simulink model "sim_motor"  (R2022b)
settings: Solver=VariableStepAuto  StartTime=0.0  StopTime=3  RelTol=1e-3
libraries: spsControlledVoltageSourceLib x1, spsDCMachineLib x1, spsDCVoltageSourceLib x1, fuzblock x1, spspowerguiLib x1
settings Model: Creator=alwal  LastModifiedBy=alwal
settings DataIOCC: SaveOutput=off  SaveTime=off  ReturnWorkspaceOutputs=off

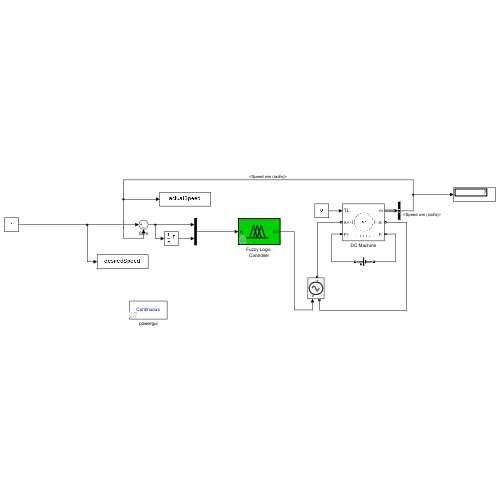
[thumbnail: Simulink's stored preview of the top-level diagram]
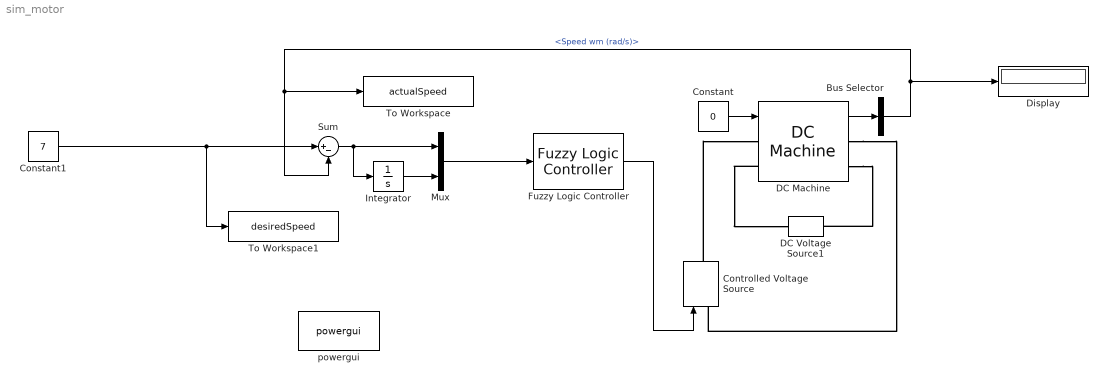
== system sim_motor ==
  Bus Selector : BusSelector  OutputSignals=Speed wm (rad/s)
  Constant : Constant  Value=0
  Constant1 : Constant  Value=7
  Controlled Voltage Source : spsControlledVoltageSourceLib/Controlled Voltage Source  Initialize=off  Source_Type=DC  Amplitude=0  Phase=0  Frequency=0  Measurements=Voltage
  DC Machine : spsDCMachineLib/DC Machine  PresetModel=No  MechanicalLoad=Torque TL  FieldType=Wound  ShowDetailedParameters=on  MeasurementBus=off  RLa="[ 0.6  0.012]"  RLf="[ 240  120]"  Laf=1.8  MachineConstant=Torque constant (N.m/A)  Ke=1.8  Kt=1.8  J=1  Bm=0  Tf=0  w0=1  Ifinit=0.0833333333333333  TsPowergui=0  TsBlock=-1
  DC Voltage Source1 : spsDCVoltageSourceLib/DC Voltage Source  Amplitude=20  Measurements=Voltage
  Display : Display
  Fuzzy Logic Controller : fuzblock/Fuzzy Logic  Controller  FIS=CLF02  OutputSampleNumber=101  DataType=double  FuzzifiedInputs=off  RuleFiringStrengths=off  RuleOutputs=off  AggregatedOutputs=off  SimulateUsing=Interpreted execution  OutOfRangeInputValueMessage=none  NoRuleFiredMessage=none  EmptyOutputFuzzySetMessage=none
  Integrator : Integrator  LimitOutput=on  UpperSaturationLimit=[9.7]  LowerSaturationLimit=[-9.7]
  Mux : Mux  Inputs=2
  Sum : Sum  Inputs=|+-
  To Workspace : ToWorkspace  VariableName=actualSpeed  SaveFormat=Timeseries
  To Workspace1 : ToWorkspace  VariableName=desiredSpeed  SaveFormat=Timeseries
  powergui : spspowerguiLib/powergui  Priority=1  SimulationMode=Continuous  SampleTime=50e-6  frequency=60  Iterations=50  frequencyindice=0  Pbase=100e6  ErrMax=1e-4  UnitsV=kV  UnitsW=MW  buscounter=0  FunctionMessages=off  echomessages=off  EnableUseOfTLC=off  CurrentSourceSwitches=off  DisableSnubberDevices=off  DisableRonSwitches=off  DisableVfSwitches=off  DisplayEquations=off  AutomaticDiscreteSolvers=off  SolverType=Tustin/Backward Euler (TBE)  Interpol=off  ExternalGateDelay=off  methode=off  Ts=100  x0status=blocks  SPID=on  SwTol=0  HookPort=off  NonlinearTolerance=1e-4  nMaxIteration=100  ContinueOnMaxIteration=off  RestoreLinks=warning  ResistiveCurrentMeasurement=off  Frange=[0:2:500]  Ylog=off  Xlog=on  ShowGrid=off  save=off  variable=ZData  structure=0  ZoomFFT=off  StartTime=0.0  cycles=1  DisplayStyle=1  fundamental=60  FreqAxis=off  MaxFrequency=1000  frequencyindicesteady=1  RmsSteady=1  display=off
  wires:
  Constant/1 -> DC Machine/1
  Bus Selector/1 -> Display/1, Sum/2, To Workspace/1  "<Speed wm (rad/s)>"
  DC Machine/1 -> Bus Selector/1
  Constant1/1 -> Sum/1, To Workspace1/1
  Integrator/1 -> Mux/2
  Sum/1 -> Mux/1, Integrator/1
  Fuzzy Logic Controller/1 -> Controlled Voltage Source/1
  Mux/1 -> Fuzzy Logic Controller/1
  connections:
  Controlled Voltage Source/RConn1 -- DC Machine/LConn1
  DC Machine/RConn1 -- Controlled Voltage Source/LConn1
  DC Machine/LConn2 -- DC Voltage Source1/RConn1
  DC Machine/RConn2 -- DC Voltage Source1/LConn1
